simulink model "plc_coder_support"  (R2025b)
settings: Solver=FixedStepDiscrete  StartTime=0.0  StopTime=30  FixedStep=0.1  RelTol=1e-3
libraries: SignalEditorBlockLib x1
settings Model: Creator=common  LastModifiedBy=KoayXianCong
settings ConfigComp: PLC_TargetIDE=gxworks3  PLC_GenerateTestbench=on  PLC_GenerateTestbenchDiagCode=on  PLC_MultiTBSigbuilderTimeRange=off  PLC_FoldFBCallOutputVar=off  PLC_RemoveUnusedSSMethodCallArguments=off  PLC_UseCallOutputArgSyntax=off  PLC_EnableUnsignedAndDoubleTypes=off  PLC_EnableUDTSplitting=off  PLC_MaxFieldsInUDT=500.0  PLC_InlineEnumCastFunction=off  PLC_RTWMaxIdLength=31.0  PLC_RollThreshold=5.0  PLC_AbsTimeTemporalLogic=counter  PLC_ActiveTab=0.0  PLC_EnableStringLiteralTB=on  PLC_Enable64bitIntSupport=off

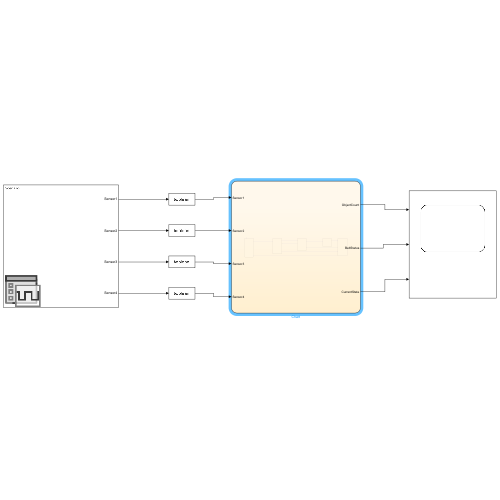
[thumbnail: Simulink's stored preview of the top-level diagram]
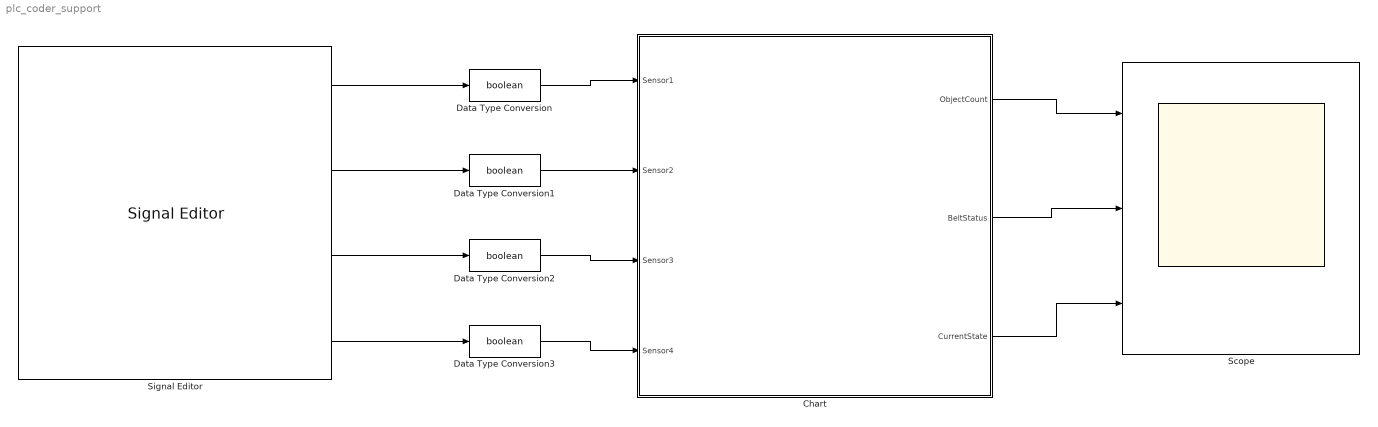
== system plc_coder_support ==
  Chart : Stateflow chart  TreatAsAtomicUnit=on
  Data Type Conversion{,1..3} (4 alike) : DataTypeConversion  OutDataTypeStr=boolean  SaturateOnIntegerOverflow=off  RndMeth=Floor
  Scope : Scope  NumInputPorts=3
      settings: TimeSpan=70  ActiveDisplayYMinimum=0
  Signal Editor : SignalEditorBlockLib/Signal Editor  FileName=ConveyorSensors.mat  ActiveScenario=Scenario  ActiveSignal=Sensor1  IsBus=off  OutputBusObjectStr=Bus: BusObject  SampleTime=0  Interpolate=off  ZeroCross=off  OutputAfterFinalValue=Setting to zero  Unit=inherit  PreserveSignalName=on  ApplySigPropsToAllScenarios=on  ApplySigPropsToAllSignals=off  SignalPropertySource=Dialog parameters
  wires:
  Signal Editor/3 -> Data Type Conversion2/1
  Data Type Conversion2/1 -> Chart/3(Sensor3)
  Chart/3(CurrentState) -> Scope/3
  Data Type Conversion1/1 -> Chart/2(Sensor2)
  Signal Editor/1 -> Data Type Conversion/1
  Data Type Conversion/1 -> Chart/1(Sensor1)
  Chart/2(BeltStatus) -> Scope/2
  Signal Editor/4 -> Data Type Conversion3/1
  Data Type Conversion3/1 -> Chart/4(Sensor4)
  Signal Editor/2 -> Data Type Conversion1/1
  Chart/1(ObjectCount) -> Scope/1

== stateflow chart plc_coder_support/Chart ==
  settings: updateMethod=DISCRETE  sampleTime=0.1
  state IDLE
    entry:
    BeltStatus = false;
    CurrentState = 0;
    objectInSystem = false;
    during:
    if (Sensor1 == true && Sensor1Previous == false)
    ObjectCount = ObjectCount + 1;
    end
    Sensor1Previous = Sensor1;
  state MOVING_TO_SENSOR2
    entry:
    BeltStatus = true;
    CurrentState = 1;
    objectInSystem = true;
    during:
    if (Sensor1 == true && Sensor1Previous == false)
    ObjectCount = ObjectCount + 1;
    end
    Sensor1Previous = Sensor1;
  state WAITING_AT_SENSOR2
    entry:
    BeltStatus = false;
    CurrentState = 2;
    during:
    if (Sensor1 == true && Sensor1Previous == false)
    ObjectCount = ObjectCount + 1;
    end
    Sensor1Previous = Sensor1;
  state MOVING_TO_SENSOR4
    entry:
    BeltStatus = true;
    CurrentState = 3;
    during:
    if (Sensor1 == true && Sensor1Previous == false)
    ObjectCount = ObjectCount + 1;
    end
    Sensor1Previous = Sensor1;
  state STOPPED_AT_SENSOR4
    entry:
    BeltStatus = false;
    CurrentState = 4;
    during:
    if (Sensor1 == true && Sensor1Previous == false)
    ObjectCount = ObjectCount + 1;
    end
    Sensor1Previous = Sensor1;
  (default) -> IDLE : { ObjectCount = 0; BeltStatus = false; CurrentState = 0; Sensor1Previous = false;objectInSystem = false; }
  MOVING_TO_SENSOR2 -> WAITING_AT_SENSOR2 [order 1] : [Sensor2 == true && Sensor4 == false]
  MOVING_TO_SENSOR4 -> STOPPED_AT_SENSOR4 : [Sensor4 == true]
  WAITING_AT_SENSOR2 -> MOVING_TO_SENSOR4 [order 2] : [Sensor3 == true && after(3, sec) && Sensor4 == false && ObjectCount == 1]
  IDLE -> MOVING_TO_SENSOR2 : [Sensor1 == true && Sensor2 == false && Sensor4 == false && objectInSystem == false]
  WAITING_AT_SENSOR2 -> MOVING_TO_SENSOR2 [order 1] : [Sensor3 == true && after(3, sec) && Sensor4 == false && ObjectCount > 1]
  STOPPED_AT_SENSOR4 -> WAITING_AT_SENSOR2 [order 1] : [Sensor4 == false && after(3, sec) && ObjectCount > 1]{ObjectCount = ObjectCount - 1; objectInSystem = true;}
  MOVING_TO_SENSOR2 -> STOPPED_AT_SENSOR4 [order 2] : [Sensor2 == true && Sensor4 == true]
  STOPPED_AT_SENSOR4 -> IDLE [order 2] : [Sensor4 == false && after(3, sec) && ObjectCount == 1]{ObjectCount = ObjectCount - 1; BeltStatus = false; CurrentState = 0; objectInSystem = false;}
  data: Sensor1 input boolean size=1; Sensor2 input boolean size=1; Sensor3 input boolean size=1; Sensor4 input boolean size=1; ObjectCount output uint32 size=1 =0; BeltStatus output boolean size=1 =0; Sensor1Previous local boolean size=1 =0; CurrentState output uint32 size=1 =0; objectInSystem local boolean size=1 =0
